simulink model "PIDEstimator"  (Simulink 10.0)
settings: Solver=ode3  StartTime=0.0  StopTime=Tsim  FixedStep=deltat  RelTol=1e-3  EnableMultiTasking=on
values from neighbouring files (symbols this model uses):
  a0 = 0.01    [Q5.m]    (also in main3.m = 1; param3.m = -1)
  a1 = 0.2    [Q5.m]    (also in main3.m = 0; param3.m = 0)
  alpha3 = 4    [main3.m]    (also in param3.m)
  dAmp = 20    [Sol_Q1.m]    (also in main3.m = -3; param3.m = -2)
  deltat = 0.01    [Q4.m]    (also in Sol_Q1.m = 0.001; main3.m; param3.m = 0.001; params2.m = 0.1)
  Gs = tf(b, [1 a])    [Q4.m]    (also in Q5.m = tf([b1 b0], [1 a1 a0]); Sol_Q1.m = tf(num, den); main3.m = tf(num, den); param3.m = tf(b, [1 a1 a0]))
  K1 = (alpha1 - a)/b    (= 1.5)    [Q4.m]    (also in Sol_Q1.m = 5; main3.m = 4; param3.m = 5)
  K2 = alpha2/b    (= 15)    [Sol_Q1.m]    (also in main3.m = 2.121; param3.m = 2.121)
  K3 = alpha3/b    (= 2)    [main3.m]    (also in param3.m)
  tauf = 0.1*tauD    (= 0.053025)    [main3.m]    (also in param3.m = 0.04242)
  Tsim = 20    [Sol_Q1.m]    (also in main3.m = 10)
  umax = 8.8    [Q4.m]    (also in Sol_Q1.m = 10000; main3.m = 4.5; param3.m = 999)
  umin = -100    [Q4.m]    (also in Sol_Q1.m = -10000; main3.m = -0.9; param3.m = -999)
settings Model: Creator=e50128  LastModifiedBy=adityaaaap
settings DataIOCC: LimitDataPoints=on  SignalLoggingSaveFormat=ModelDataLogs
settings OptimizationCC: ExpressionDepthLimit=2147483647
settings DebuggingCC: SolverPrmCheckMsg=warning  FcnCallInpInsideContextMsg=warning  StateNameClashWarn=warning
settings GRTTargetCC: GeneratePreprocessorConditionals=Disable all
settings ConfigComp: CovExternalEMLEnable=off

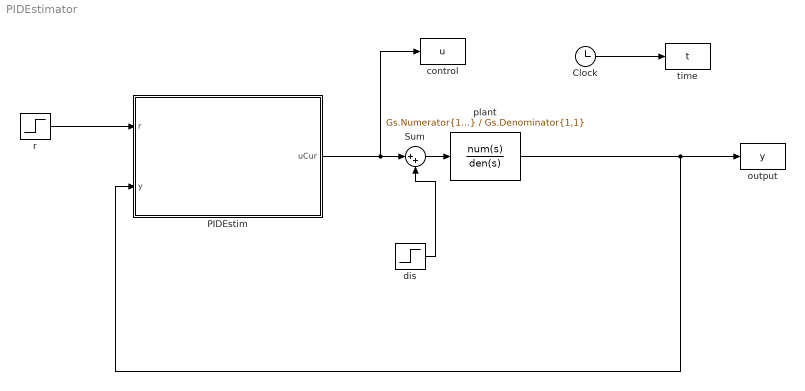
== system PIDEstimator ==
  Clock : Clock
  PIDEstim : MATLAB Function  TreatAsAtomicUnit=on
  Sum : Sum  Inputs=|++
  control : ToWorkspace  VariableName=u
      settings: MaxDataPoints=10000
  dis : Step  Time=Tsim/2  After=dAmp  SampleTime=0
  output : ToWorkspace  VariableName=y
      settings: MaxDataPoints=10000
  plant : TransferFcn  Numerator=Gs.Numerator{1,1}  Denominator=Gs.Denominator{1,1}
  r : Step  Time=0  SampleTime=0
  time : ToWorkspace  VariableName=t
      settings: MaxDataPoints=10000
  wires:
  r/1 -> PIDEstim/1(r)
  Clock/1 -> time/1
  plant/1 -> output/1, PIDEstim/2(y)
  PIDEstim/1(uCur) -> control/1, Sum/1
  dis/1 -> Sum/2
  Sum/1 -> plant/1

== matlab function PIDEstim ==
  settings: updateMethod=DISCRETE  sampleTime=deltat
  data: uCur output double; r input double; y input double; K1 parameter double; K2 parameter double; K3 parameter double; tauf parameter double; alpha3 parameter double; a1 parameter double; a0 parameter double; deltat parameter double; umin parameter double; umax parameter double
function uCur = PIDEstFD(r,y,K1,K2,K3,tauf,alpha3,a1,a0,deltat,umin,umax)
persistent zhat
if isempty(zhat)
    zhat=0;
end
persistent ydfpast
if isempty(ydfpast)
    ydfpast=0;
end
persistent ypast
if isempty(ypast)
    ypast=0;
end


% ndmax=100; 
% persistent(udelay)
% if isempty(udelay)
%     udelay=zeros(1,ndmax);
% end   
%estimator based MATLAB function with anti-windup
ydf=tauf/(tauf+deltat)*ydfpast+1/(tauf+deltat)*(y-ypast); 
dhat=zhat+K3*ydf;   
uCur= -K1*(y-r)-K2*ydf-dhat;
if (uCur>umax) uCur=umax;end
if (uCur<umin) uCur=umin;end
zhat=zhat-deltat*alpha3*zhat+deltat*(K3*(a1-alpha3)*ydf+K3*a0*(y-r)-alpha3*uCur);
ypast=y;
ydfpast=ydf;
%udelay=[uCur udelay(1,1:ndmax-1)];
